simulink model "AxleSplitHEVv6_modif2019"  (R2018b)
settings: Solver=ode5  StartTime=0.0  StopTime=400  FixedStep=hev_dt  MaxStep=0.01  RelTol=1e-3  AbsTol=1e-3  EnableMultiTasking=on
PostLoadFcn:
  | load('AxelSplitHEVv4_NEDC_18_06_15.mat')
values from neighbouring files (symbols this model uses):
  cmd_equivalent_conso_coef = 0.11126984    [AxelSplitHEVv4_NEDC_18_06_15.mat]
  cmd_qmax = 42    [AxelSplitHEVv4_NEDC_18_06_15.mat]
  cmd_specific_volume_l_per_g = 0.00133333333333    [AxelSplitHEVv4_NEDC_18_06_15.mat]
  dri_cycle_speed_sp = [0 0 0 4.16666667 4.16666667 2.777777778 0 0 0 4.166666667 4.166666667 8.88888889 ... (135 elements, 135x1)]    [AxelSplitHEVv4_NEDC_18_06_15.mat]
  dri_cycle_speed_time = [0 6 11 15 23 25 28 44 49 54 56 61 ... (135 elements, 135x1)]    [AxelSplitHEVv4_NEDC_18_06_15.mat]
  dri_gbx_sp = [0 1 0 1 2 0 1 2 3 2 0 1 ... (52 elements, 52x1)]    [AxelSplitHEVv4_NEDC_18_06_15.mat]
  dri_gbx_time = [0 11 25 49 55 93 117 123 134 177 185 206 ... (52 elements, 52x1)]    [AxelSplitHEVv4_NEDC_18_06_15.mat]
  dri_ki = 24.5    [AxelSplitHEVv4_NEDC_18_06_15.mat]
  dri_kp = 609    [AxelSplitHEVv4_NEDC_18_06_15.mat]
  fa_clu_pos = [1 1 0.7 0.5 0.3 0 0]    [AxelSplitHEVv4_NEDC_18_06_15.mat]
  fa_clu_pv = [0 0.1 0.3 0.5 0.7 0.9 1]    [AxelSplitHEVv4_NEDC_18_06_15.mat]
  fa_conso_idle = 0.153611111111    [AxelSplitHEVv4_NEDC_18_06_15.mat]
  fa_conso_speed = [200 300 400 500 600 700 800 900 1000 1100 1200 1300 ... (56 elements, 1x56)]    [AxelSplitHEVv4_NEDC_18_06_15.mat]
  fa_conso_torque = [0 6.66666666667 13.3333333333 20 26.6666666667 33.3333333333 40 46.6666666667 53.3333333333 60 66.6666666667 73.3333333333 ... (43 elements, 1x43)]    [AxelSplitHEVv4_NEDC_18_06_15.mat]
  fa_delta_derating = 500    [AxelSplitHEVv4_NEDC_18_06_15.mat]
  fa_differential_ratio = FDR.fa_differential_ratio    [Algorithme_eff.m]    (also in AxelSplitHEVv4_NEDC_18_06_15.mat = 3.72; fa_differential_ratio.mat = 3.72)
  fa_fuel_consumption = [nan nan nan nan nan nan nan nan nan nan nan nan ... (2408 elements, 43x56)]    [AxelSplitHEVv4_NEDC_18_06_15.mat]    (also in Curve_fitting_conso.m = fa_fuel_consumption/max(max(fa_fuel_consumption)))
  fa_gearbox_efficiency = 0.92    [AxelSplitHEVv4_NEDC_18_06_15.mat]
  fa_gearbox_ratio = FGR.fa_gearbox_ratio    [Algorithme_eff.m]    (also in AxelSplitHEVv4_NEDC_18_06_15.mat = [0 3.98 2.21 1.47 1.1 0.89 0.75]; fa_gearbox_ratio.mat = [0 3.98 2.21 1.47 1.1 0.89 0.75])
  fa_high_derating_point = 5700    [AxelSplitHEVv4_NEDC_18_06_15.mat]
  fa_ice_inertia = 0.058    [AxelSplitHEVv4_NEDC_18_06_15.mat]
  fa_kp_idle_tr_off = 0.116198282851    [AxelSplitHEVv4_NEDC_18_06_15.mat]
  fa_kp_idle_tr_on = [1 0.8653 2.8063 6.3428 11.3274 17.3036 24.3665]    [AxelSplitHEVv4_NEDC_18_06_15.mat]
  fa_low_derating_point = 4000    [AxelSplitHEVv4_NEDC_18_06_15.mat]
  fa_max_tq_clu = 206    [AxelSplitHEVv4_NEDC_18_06_15.mat]
  fa_max_tq_ice = [0 220 233.333333333 240 246.666666667 253.333333333 253.333333333 253.333333333 260 260 266.666666667 266.666666667 ... (52 elements, 1x52)]    [AxelSplitHEVv4_NEDC_18_06_15.mat]
  fa_n_ice = [0 20 250 850 1000 1250 1500 1750 2000 2250 2500 3000 ... (18 elements, 1x18)]    [AxelSplitHEVv4_NEDC_18_06_15.mat]
  fa_starter_rpm = [0 10 20 30 40 50 60 70 80 90 100 110 ... (101 elements, 1x101)]    [AxelSplitHEVv4_NEDC_18_06_15.mat]
  fa_starter_tq = [24 24 24 24 23.3333333333 23.3333333333 23.3333333333 22.6666666667 22.6666666667 22 21.3333333333 20.6666666667 ... (101 elements, 1x101)]    [AxelSplitHEVv4_NEDC_18_06_15.mat]
  fa_tau_ice = 0.0333    [AxelSplitHEVv4_NEDC_18_06_15.mat]
  fa_taui_idle_tr_off = 0.0820482966067    [AxelSplitHEVv4_NEDC_18_06_15.mat]
  fa_taui_idle_tr_on = 0.194086623254    [AxelSplitHEVv4_NEDC_18_06_15.mat]
  fa_tq_loss = [0 -11 -10 -9 -9 -10 -11 -11 -12 -13 -14 -15 ... (18 elements, 1x18)]    [AxelSplitHEVv4_NEDC_18_06_15.mat]
  fa_tq_max_speed = [200 700 800 900 1000 1100 1200 1300 1400 1500 1600 1700 ... (52 elements, 1x52)]    [AxelSplitHEVv4_NEDC_18_06_15.mat]
  hev_dt = 0.01    [AxelSplitHEVv4_NEDC_18_06_15.mat]
  pla_csat = 1.2    [AxelSplitHEVv4_NEDC_18_06_15.mat]
  pla_equivalent_weight = 1250    [AxelSplitHEVv4_NEDC_18_06_15.mat]
  pla_f = 0.0035272    [AxelSplitHEVv4_NEDC_18_06_15.mat]
  pla_k = 0.0002318    [AxelSplitHEVv4_NEDC_18_06_15.mat]
  pla_kaero = 0.52992    [AxelSplitHEVv4_NEDC_18_06_15.mat]
  pla_max_f_brakes = 1000    [AxelSplitHEVv4_NEDC_18_06_15.mat]
  pla_wheel_radius = 0.314    [AxelSplitHEVv4_NEDC_18_06_15.mat]
  ra_electrical_machine_efficiency = [nan nan nan nan nan nan nan 91.3 91.3 91.3 91.5 91.3 ... (777 elements, 37x21)]    [AxelSplitHEVv4_NEDC_18_06_15.mat]
  ra_electrical_machine_speed = [-12000 -10800 -9600 -8400 -7200 -6000 -4800 -3600 -2400 -1200 0 1200 ... (21 elements, 1x21)]    [AxelSplitHEVv4_NEDC_18_06_15.mat]
  ra_electrical_machine_tau = 0.1    [AxelSplitHEVv4_NEDC_18_06_15.mat]
  ra_electrical_machine_torque = [-79.6460176991 -75.2212389381 -70.796460177 -66.3716814159 -61.9469026549 -57.5221238938 -53.0973451327 -48.6725663717 -44.2477876106 -39.8230088496 -35.3982300885 -30.9734513274 ... (37 elements, 1x37)]    [AxelSplitHEVv4_NEDC_18_06_15.mat]
  ra_em_max_tq = [39.8230088496 44.2477876106 53.0973451327 57.5221238938 70.796460177 79.6460176991 79.6460176991 79.6460176991 79.6460176991 79.6460176991 79.6460176991 79.6460176991 ... (21 elements, 1x21)]    [AxelSplitHEVv4_NEDC_18_06_15.mat]
  ra_em_min_tq = [-39.8230088496 -44.2477876106 -53.0973451327 -57.5221238938 -70.796460177 -79.6460176991 -79.6460176991 -79.6460176991 -79.6460176991 -79.6460176991 -79.6460176991 -79.6460176991 ... (21 elements, 1x21)]    [AxelSplitHEVv4_NEDC_18_06_15.mat]
  ra_transmission_efficiency = 0.92    [AxelSplitHEVv4_NEDC_18_06_15.mat]
  reducteur = 2    [Main_modif.m]
  syse_aux_current = 33.3    [AxelSplitHEVv4_NEDC_18_06_15.mat]
  syse_aux_voltage = 12    [AxelSplitHEVv4_NEDC_18_06_15.mat]
  syse_bat_nominal_capacity_as = 151200    [AxelSplitHEVv4_NEDC_18_06_15.mat]
  syse_cdl = 5000    [AxelSplitHEVv4_NEDC_18_06_15.mat]
  syse_dcdc_efficency = [78 89.6 92.5 95.2 95 94.6]    [AxelSplitHEVv4_NEDC_18_06_15.mat]
  syse_dcdc_in_power = [54 135 202 405 1485 2000]    [AxelSplitHEVv4_NEDC_18_06_15.mat]
  syse_electrical_machine_torque_vs_power_speed_nneg = [38.4209635438 42.3166718474 53.0973451327 53.8788373627 63.500986907 77.9700595469 78.3175021924 76.9635177026 72.2987813984 47.9837613501 38.4209635438 42.3166718474 ... (220 elements, 10x22)]    [AxelSplitHEVv4_NEDC_18_06_15.mat]
  syse_electrical_machine_torque_vs_power_speed_npos = [-72.2987813984 -76.9635177026 -78.3175021924 -77.9700595469 -63.500986907 -53.8788373627 -53.0973451327 -42.3166718474 -38.4209635438 -72.2987813984 -76.9635177026 -78.3175021924 ... (198 elements, 9x22)]    [AxelSplitHEVv4_NEDC_18_06_15.mat]
  syse_em_in_power = [-49.1089315336 -44.1089315336 -39.1089315336 -34.1089315336 -29.1089315336 -24.1089315336 -19.1089315336 -14.1089315336 -9.10893153364 -4.10893153364 0.891068466363 5.89106846636 ... (22 elements, 1x22)]    [AxelSplitHEVv4_NEDC_18_06_15.mat]
  syse_max_charge_current = [8.4 8.4 42 92.4 92.4 92.4 92.4 92.4 79.8 42 21 4.2]    [AxelSplitHEVv4_NEDC_18_06_15.mat]
  syse_max_discharge_current = [42 42 79.8 159.6 180.6 180.6 180.6 180.6 180.6 180.6 180.6 180.6]    [AxelSplitHEVv4_NEDC_18_06_15.mat]
  syse_nb_cell = 52    [AxelSplitHEVv4_NEDC_18_06_15.mat]
  syse_rdl = 0.004    [AxelSplitHEVv4_NEDC_18_06_15.mat]
  syse_rser = 0.002    [AxelSplitHEVv4_NEDC_18_06_15.mat]
  syse_soc_current_limits = [0 10 20 20.1 30 40 50 60 70 80 90 100]    [AxelSplitHEVv4_NEDC_18_06_15.mat]
  syse_soc_initial = 0.8    [AxelSplitHEVv4_NEDC_18_06_15.mat]
  syse_soc_ocv = [0 5 10 20 40 50 60 70 80 90 100]    [AxelSplitHEVv4_NEDC_18_06_15.mat]
  syse_vocv = [2.5 3.2135 3.5127 3.66 3.7771 3.8181 3.8686 3.8978 3.9429 4.0006 4.198]    [AxelSplitHEVv4_NEDC_18_06_15.mat]
undefined symbols (not defined in the file or in its folder): DiscIntNeverNeededParam
libraries: simulink x23, simulink_extras x1
(part 1 of 3)
settings Model: Creator=jboursie  LastModifiedBy=test
settings SolverCC: AutoScaleAbsTol=off  AlgebraicLoopSolver=LineSearch
settings DataIOCC: SaveFormat=Array  SignalLoggingSaveFormat=ModelDataLogs  SaveOutput=off  SignalLogging=off  DSMLogging=off  SaveTime=off
settings OptimizationCC: LifeSpan=inf
settings DebuggingCC: AlgebraicLoopMsg=error  UnderspecifiedInitializationDetection=Classic  MergeDetectMultiDrivingBlocksExec=none  SolverPrmCheckMsg=warning  MultiTaskCondExecSysMsg=none  MultiTaskRateTransMsg=warning  FcnCallInpInsideContextMsg=warning  BusObjectLabelMismatch=error  StateNameClashWarn=warning  SFUnexpectedBacktrackingDiag=warning  SFNoUnconditionalDefaultTransitionDiag=warning  SFExecutionAtInitializationDiag=none
settings HardwareCC: ProdBitPerPointer=32  ProdBitPerSizeT=32  ProdBitPerPtrDiffT=32  ProdLargestAtomicFloat=None  ProdIntDivRoundTo=Undefined  ProdEndianess=Unspecified  ProdWordSize=32  ProdHWDeviceType=32-bit Generic
settings ModelReferenceCC: PropagateSignalLabelsOutOfModel=off
settings SFSimCC: SimUseLocalCustomCode=off
settings RTWCC: RTWUseLocalCustomCode=off
settings CodeAppCC: StateflowObjectComments=on
settings GRTTargetCC: TargetLangStandard=C89/C90 (ANSI)  GeneratePreprocessorConditionals=Disable all  CombineOutputUpdateFcns=off  GRTInterface=on
settings ConfigComp: CovMetricSettings=dw  CovHtmlReporting=on  CovSaveCumulativeToWorkspaceVar=on  CovSaveSingleToWorkspaceVar=on  CovExternalEMLEnable=off

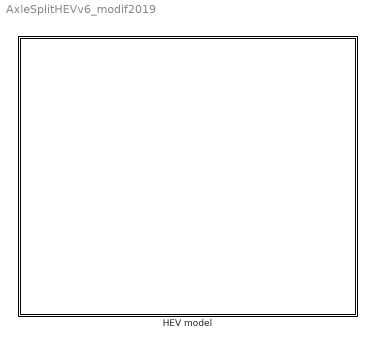
== system AxleSplitHEVv6_modif2019 ==
  HEV model : Subsystem

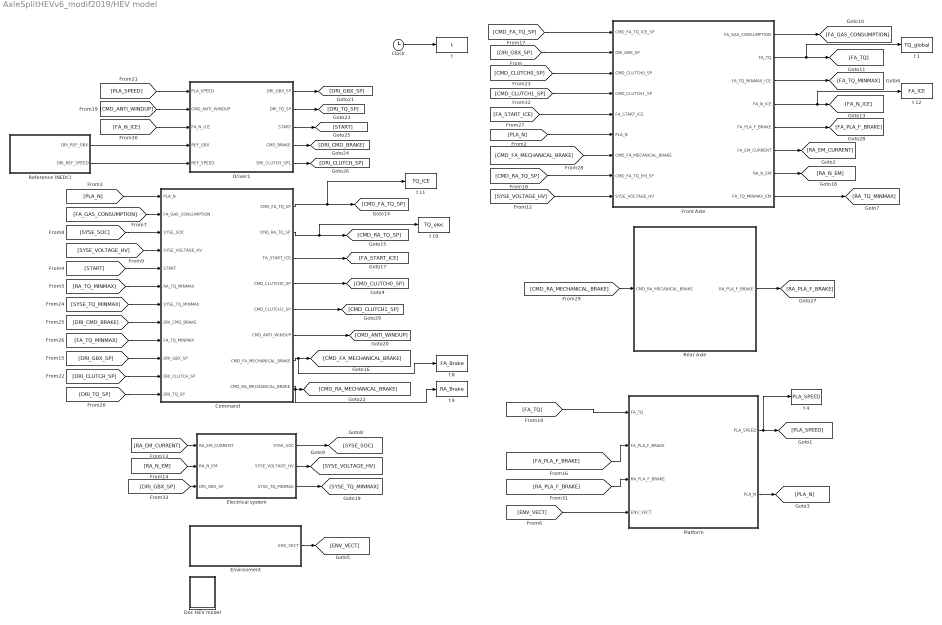
== system AxleSplitHEVv6_modif2019/HEV model ==
  Clock : Clock
  Command : Subsystem
  Doc HEV model : Subsystem
      settings: OpenFcn=open('Documents\HEVmodel.pdf')
      mask Display: fprintf('DOC')
  Driver1 : Subsystem
  Electrical system : Subsystem
  Environment : Subsystem
  Front Axle : Subsystem
  Platform : Subsystem
  Rear Axle : Subsystem
  Reference (NEDC) : Subsystem
  "t " : ToWorkspace  VariableName=t  SampleTime=hev_dt
  t 1 : ToWorkspace  VariableName=TQ_global  SampleTime=hev_dt
  t 10 : ToWorkspace  VariableName=TQ_elec  SampleTime=hev_dt
  t 11 : ToWorkspace  VariableName=TQ_ICE  SampleTime=hev_dt
  t 12 : ToWorkspace  VariableName=FA_ICE  SampleTime=hev_dt
  t 4 : ToWorkspace  VariableName=PLA_SPEED  SampleTime=hev_dt
  t 8 : ToWorkspace  VariableName=FA_Brake  SampleTime=hev_dt
  t 9 : ToWorkspace  VariableName=RA_Brake  SampleTime=hev_dt
  wires:
  Environment/1(ENV_VECT) -> [ENV_VECT]
  Electrical system/2(SYSE_VOLTAGE_HV) -> [SYSE_VOLTAGE_HV]
  Electrical system/1(SYSE_SOC) -> [SYSE_SOC]
  [RA_EM_CURRENT] -> Electrical system/1(RA_EM_CURRENT)
  [RA_N_EM] -> Electrical system/2(RA_N_EM)
  Electrical system/3(SYSE_TQ_MINMAX) -> [SYSE_TQ_MINMAX]
  Clock/1 -> "t "/1
  [CMD_ANTI_WINDUP] -> Driver1/2(CMD_ANTI_WINDUP)
  Driver1/1(DRI_GBX_SP) -> [DRI_GBX_SP]
  Driver1/2(DRI_TQ_SP) -> [DRI_TQ_SP]
  Driver1/5(DRI_CLUTCH_SP1) -> [DRI_CLUTCH_SP]
  Driver1/3(START) -> [START]
  Driver1/4(CMD_BRAKE) -> [DRI_CMD_BRAKE]
  [FA_N_ICE] -> Driver1/3(FA_N_ICE)
  Reference (NEDC)/2(DRI_REF_SPEED) -> Driver1/5(REF_SPEED)
  Reference (NEDC)/1(DRI_REF_GBX) -> Driver1/4(REF_GBX)
  [PLA_SPEED] -> Driver1/1(PLA_SPEED)
  [PLA_N] -> Command/1(PLA_N)
  [RA_TQ_MINMAX] -> Command/6(RA_TQ_MINMAX)
  [FA_GAS_CONSUMPTION] -> Command/2(FA_GAS_CONSUMPTION)
  [SYSE_SOC] -> Command/3(SYSE_SOC)
  [SYSE_VOLTAGE_HV] -> Command/4(SYSE_VOLTAGE_HV)
  Command/2(CMD_RA_TQ_SP) -> t 10/1, [CMD_RA_TQ_SP]
  Command/7(CMD_FA_MECHANICAL_BRAKE) -> t 8/1, [CMD_FA_MECHANICAL_BRAKE]
  [DRI_TQ_SP] -> Command/12(DRI_TQ_SP)
  [DRI_CLUTCH_SP] -> Command/11(DRI_CLUTCH_SP)
  [DRI_GBX_SP] -> Command/10(DRI_GBX_SP)
  [SYSE_TQ_MINMAX] -> Command/7(SYSE_TQ_MINMAX)
  [START] -> Command/5(START)
  Command/3(FA_START_ICE) -> [FA_START_ICE]
  [DRI_CMD_BRAKE] -> Command/8(DRI_CMD_BRAKE)
  [FA_TQ_MINMAX] -> Command/9(FA_TQ_MINMAX)
  Command/4("CMD_CLUTCH0_SP ") -> [CMD_CLUTCH0_SP]
  Command/6(CMD_ANTI_WINDUP) -> [CMD_ANTI_WINDUP]
  Platform/1(PLA_SPEED) -> t 4/1, [PLA_SPEED]
  Platform/2(PLA_N) -> [PLA_N]
  Front Axle/3(FA_TQ_MINMAX_ICE) -> [FA_TQ_MINMAX]
  Front Axle/8(FA_TQ_MINMAX_EM) -> [RA_TQ_MINMAX]
  [ENV_VECT] -> Platform/4(ENV_VECT)
  Front Axle/1(FA_GAS_CONSUMPTION) -> [FA_GAS_CONSUMPTION]
  Front Axle/2(FA_TQ) -> t 1/1, [FA_TQ]
  [FA_TQ] -> Platform/1(FA_TQ)
  [SYSE_VOLTAGE_HV] -> Front Axle/9(SYSE_VOLTAGE_HV)
  Front Axle/6(FA_EM_CURRENT) -> [RA_EM_CURRENT]
  [FA_PLA_F_BRAKE] -> Platform/2(FA_PLA_F_BRAKE)
  [CMD_RA_TQ_SP] -> Front Axle/8(CMD_FA_TQ_EM_SP)
  Front Axle/7(RA_N_EM) -> [RA_N_EM]
  [PLA_N] -> Front Axle/6(PLA_N)
  [FA_START_ICE] -> Front Axle/5(FA_START_ICE)
  [DRI_GBX_SP] -> Front Axle/2(DRI_GBX_SP)
  [CMD_CLUTCH0_SP] -> Front Axle/3(CMD_CLUTCH0_SP)
  Front Axle/4(FA_N_ICE) -> t 12/1, [FA_N_ICE]
  [CMD_FA_TQ_SP] -> Front Axle/1(CMD_FA_TQ_ICE_SP)
  [CMD_FA_MECHANICAL_BRAKE] -> Front Axle/7(CMD_FA_MECANICAL_BRAKE)
  [CMD_RA_MECHANICAL_BRAKE] -> Rear Axle/1(CMD_RA_MECANICAL_BRAKE)
  [RA_PLA_F_BRAKE] -> Platform/3(RA_PLA_F_BRAKE)
  Rear Axle/1(RA_PLA_F_BRAKE) -> [RA_PLA_F_BRAKE]
  Front Axle/5(FA_PLA_F_BRAKE) -> [FA_PLA_F_BRAKE]
  Command/8(CMD_RA_MECHANICAL_BRAKE) -> t 9/1, [CMD_RA_MECHANICAL_BRAKE]
  Command/1(CMD_FA_TQ_SP) -> t 11/1, [CMD_FA_TQ_SP]
  [CMD_CLUTCH1_SP] -> Front Axle/4(CMD_CLUTCH1_SP)
  Command/5("CMD_CLUTCH1_SP ") -> [CMD_CLUTCH1_SP]
  [DRI_GBX_SP] -> Electrical system/3(DRI_GBX_SP)

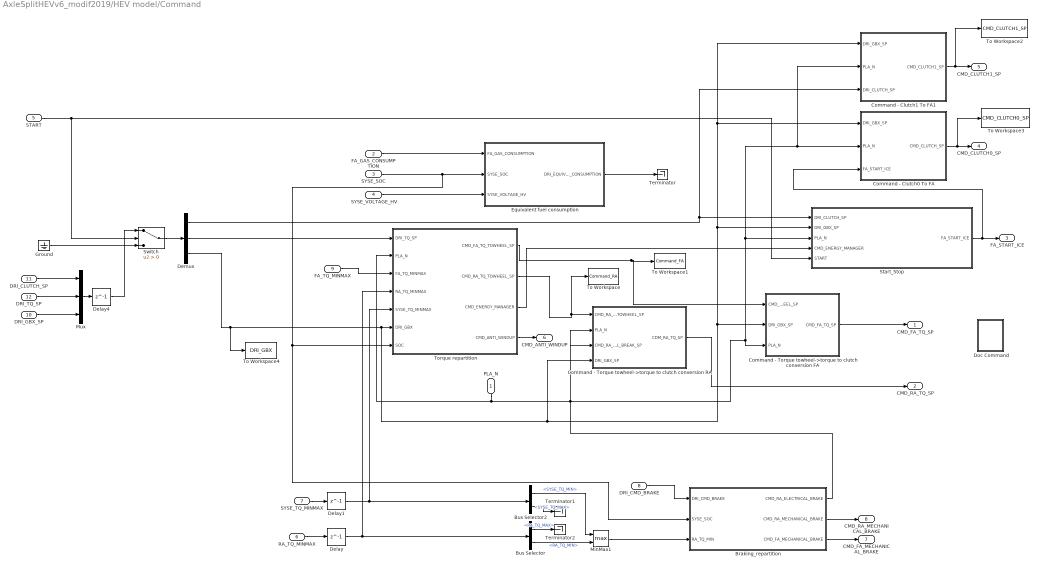
== system AxleSplitHEVv6_modif2019/HEV model/Command ==
  PLA_N : Inport
  FA_GAS_CONSUMPTION : Inport  Port=2
  SYSE_SOC : Inport  Port=3
  SYSE_VOLTAGE_HV : Inport  Port=4
  START : Inport  Port=5
  RA_TQ_MINMAX : Inport  Port=6
  SYSE_TQ_MINMAX : Inport  Port=7
  DRI_CMD_BRAKE : Inport  Port=8
  FA_TQ_MINMAX : Inport  Port=9
  DRI_GBX_SP : Inport  Port=10
  DRI_CLUTCH_SP : Inport  Port=11
  DRI_TQ_SP : Inport  Port=12
  Braking_repartition : Subsystem
  Bus Selector : BusSelector  OutputSignals=RA_TQ_MAX,RA_TQ_MIN
  Bus Selector2 : BusSelector  OutputSignals=SYSE_TQ_MIN,SYSE_TQ_MAX
  Command - Clutch0 To FA : Subsystem
  Command - Clutch1 To FA1 : Subsystem
  Command - Torque towheel->torque to clutch conversion FA : Subsystem
  Command - Torque towheel->torque to clutch conversion RA : Subsystem
  Delay : Delay  DelayLength=1
  Delay1 : Delay  DelayLength=1
  Delay4 : Delay  DelayLength=1
  Demux : Demux  Outputs=3
  Doc Command : Subsystem
      settings: OpenFcn=open('Documents\Command.pdf')
      mask Display: fprintf('DOC')
  Equivalent fuel consumption : Subsystem
  Ground : Ground
  MinMax1 : MinMax  Function=max  Inputs=2  SampleTime=hev_dt
  Mux : Mux  Inputs=3
  Start_Stop : Subsystem
  Switch : Switch  Criteria=u2 > Threshold
  Terminator : Terminator
  Terminator1 : Terminator
  Terminator2 : Terminator
  To Workspace : ToWorkspace  VariableName=Command_RA  SampleTime=-1
  To Workspace1 : ToWorkspace  VariableName=Command_FA  SampleTime=-1
  To Workspace2 : ToWorkspace  VariableName=CMD_CLUTCH1_SP  SampleTime=-1
  To Workspace3 : ToWorkspace  VariableName=CMD_CLUTCH0_SP  SampleTime=-1
  To Workspace4 : ToWorkspace  VariableName=DRI_GBX  SampleTime=-1
  Torque repartition : Subsystem
  CMD_FA_TQ_SP : Outport
  CMD_RA_TQ_SP : Outport  Port=2
  FA_START_ICE : Outport  Port=3
  "CMD_CLUTCH0_SP " : Outport  Port=4
  "CMD_CLUTCH1_SP " : Outport  Port=5
  CMD_ANTI_WINDUP : Outport  Port=6
  CMD_FA_MECHANICAL_BRAKE : Outport  Port=7
  CMD_RA_MECHANICAL_BRAKE : Outport  Port=8
  wires:
  FA_GAS_CONSUMPTION/1 -> Equivalent fuel consumption/1(FA_GAS_CONSUMPTION)
  SYSE_SOC/1 -> Equivalent fuel consumption/2(SYSE_SOC), Braking_repartition/2(SYSE_SOC), Torque repartition/7(SOC)
  SYSE_VOLTAGE_HV/1 -> Equivalent fuel consumption/3(SYSE_VOLTAGE_HV)
  Torque repartition/1(CMD_FA_TQ_TOWHEEL_SP) -> To Workspace1/1, Command - Torque towheel->torque to clutch conversion FA/1(CMD_FA_TQ_TOWHEEL_SP)
  Equivalent fuel consumption/1(DRI_EQUIV_GAZ_CONSUMPTION) -> Terminator/1
  Command - Torque towheel->torque to clutch conversion FA/1(CMD_FA_TQ_SP) -> CMD_FA_TQ_SP/1
  RA_TQ_MINMAX/1 -> Delay/1
  SYSE_TQ_MINMAX/1 -> Delay1/1
  Bus Selector2/1 -> MinMax1/1  "<SYSE_TQ_MIN>"
  Bus Selector/2 -> MinMax1/2  "<RA_TQ_MIN>"
  Bus Selector/1 -> Terminator2/1  "<RA_TQ_MAX>"
  Bus Selector2/2 -> Terminator1/1  "<SYSE_TQ_MAX>"
  Command - Torque towheel->torque to clutch conversion RA/1(CDM_RA_TQ_SP) -> CMD_RA_TQ_SP/1
  Torque repartition/2(CMD_RA_TQ_TOWHEEL_SP) -> Command - Torque towheel->torque to clutch conversion RA/1(CMD_RA_TQ_TOWHEEL_SP), To Workspace/1
  START/1 -> Start_Stop/5(START), Switch/2
  Start_Stop/1(FA_START_ICE) -> Command - Clutch0 To FA/3(FA_START_ICE), FA_START_ICE/1
  DRI_CMD_BRAKE/1 -> Braking_repartition/1(DRI_CMD_BRAKE)
  MinMax1/1 -> Braking_repartition/3(RA_TQ_MIN)
  FA_TQ_MINMAX/1 -> Torque repartition/3(FA_TQ_MINMAX)
  Delay/1 -> Bus Selector/1, Torque repartition/4(RA_TQ_MINMAX)
  Delay1/1 -> Bus Selector2/1, Torque repartition/5(SYSE_TQ_MINMAX)
  PLA_N/1 -> Command - Torque towheel->torque to clutch conversion RA/2(PLA_N), Start_Stop/3(PLA_N), Command - Clutch1 To FA1/2(PLA_N), Command - Clutch0 To FA/2(PLA_N), Command - Torque towheel->torque to clutch conversion FA/3(PLA_N), Torque repartition/2(PLA_N)
  Command - Clutch0 To FA/1("CMD_CLUTCH_SP ") -> To Workspace3/1, "CMD_CLUTCH0_SP "/1
  Torque repartition/3(CMD_ENERGY_MANAGER) -> Start_Stop/4(CMD_ENERGY_MANAGER)
  Torque repartition/4(CMD_ANTI_WINDUP) -> CMD_ANTI_WINDUP/1
  Switch/1 -> Demux/1
  DRI_GBX_SP/1 -> Mux/3
  Mux/1 -> Delay4/1
  Demux/3 -> To Workspace4/1, Command - Torque towheel->torque to clutch conversion RA/4(DRI_GBX_SP), Start_Stop/2(DRI_GBX_SP), Command - Clutch0 To FA/1(DRI_GBX_SP), Command - Clutch1 To FA1/1(DRI_GBX_SP), Command - Torque towheel->torque to clutch conversion FA/2(DRI_GBX_SP), Torque repartition/6(DRI_GBX)
  Delay4/1 -> Switch/1
  Ground/1 -> Switch/3
  DRI_CLUTCH_SP/1 -> Mux/1
  DRI_TQ_SP/1 -> Mux/2
  Demux/2 -> Torque repartition/1(DRI_TQ_SP)
  Braking_repartition/1(CMD_RA_ELECTRICAL_BRAKE) -> Command - Torque towheel->torque to clutch conversion RA/3(CMD_RA_TQ_TOWHEEL_BREAK_SP)
  Braking_repartition/3(CMD_FA_MECHANICAL_BRAKE) -> CMD_FA_MECHANICAL_BRAKE/1
  Braking_repartition/2(CMD_RA_MECHANICAL_BRAKE) -> CMD_RA_MECHANICAL_BRAKE/1
  Command - Clutch1 To FA1/1("CMD_CLUTCH1_SP ") -> To Workspace2/1, "CMD_CLUTCH1_SP "/1
  Demux/1 -> Start_Stop/1(DRI_CLUTCH_SP), Command - Clutch1 To FA1/3(DRI_CLUTCH_SP)

== system AxleSplitHEVv6_modif2019/HEV model/Doc HEV model ==

== system AxleSplitHEVv6_modif2019/HEV model/Driver1 ==
  note: Nouvelle commande START pour éveiller le système : Le conducteur ne peut démarrer le véhicule que si START est à 1
  PLA_SPEED : Inport
  CMD_ANTI_WINDUP : Inport  Port=2
  FA_N_ICE : Inport  Port=3
  REF_GBX : Inport  Port=4
  REF_SPEED : Inport  Port=5
  Clutch command : Subsystem
  Delay : Delay  DelayLength=1
  Doc Driver : Subsystem
      settings: OpenFcn=open('Documents\Driver.pdf')
      mask Display: fprintf('DOC')
  Driver : Subsystem
  Product : Product
  Step1 : Step  Time=0  SampleTime=0
  Sum2 : Sum  Inputs=-|+  SampleTime=hev_dt
  To Workspace : ToWorkspace  VariableName=DRI_TQ  SaveFormat=Timeseries  SampleTime=-1
  DRI_GBX_SP : Outport
  DRI_TQ_SP : Outport  Port=2
  START : Outport  Port=3
  CMD_BRAKE : Outport  Port=4
  DRI_CLUTCH_SP1 : Outport  Port=5
  wires:
  CMD_ANTI_WINDUP/1 -> Driver/1(CMD_ANTI_WINDUP)
  REF_GBX/1 -> Clutch command/1(DRI_REF_GBX)
  REF_SPEED/1 -> Sum2/2  "Speed_reference_km/h"
  Driver/1(DRI_TQ_SP) -> To Workspace/1, DRI_TQ_SP/1
  Driver/2(CMD_BRAKE) -> CMD_BRAKE/1
  Sum2/1 -> Driver/2(DRI_DELTA_SPEED)
  PLA_SPEED/1 -> Sum2/1
  Step1/1 -> START/1
  FA_N_ICE/1 -> Delay/1
  Clutch command/1(DRI_GBX_SP) -> DRI_GBX_SP/1
  Clutch command/2(DRI_CLUTCH_SP) -> Product/2
  Delay/1 -> Clutch command/2(FA_N_ICE)
  Driver/3(DRI_CLUTCH) -> Product/1
  Product/1 -> DRI_CLUTCH_SP1/1

== system AxleSplitHEVv6_modif2019/HEV model/Electrical system ==
  RA_EM_CURRENT : Inport
  RA_N_EM : Inport  Port=2
  DRI_GBX_SP : Inport  Port=3
  Add : Sum  SampleTime=hev_dt
  Auxiliary network 12V : Subsystem
  Bus Creator : BusCreator  Inputs=2
  Delay : Delay  DelayLength=1  SampleTime=hev_dt
  Doc Electrical system : Subsystem
      settings: OpenFcn=open('Documents\ElectricalSystem.pdf')
      mask Display: fprintf('DOC')
  Electrical System supervision : Subsystem
  Lithium-Ion Battery Management System : Subsystem
  SYSE_SOC : Outport
  SYSE_VOLTAGE_HV : Outport  Port=2
  SYSE_TQ_MINMAX : Outport  Port=3
  wires:
  Add/1 -> Delay/1  "A"
  Lithium-Ion Battery Management System/2(SYSE_VOLTAGE_HV) -> Electrical System supervision/4(SYSE_VOLTAGE_HV), SYSE_VOLTAGE_HV/1, Auxiliary network 12V/1(SYSE_VOLTAGE_HV)  "V"
  Lithium-Ion Battery Management System/1(SYSE_SOC) -> SYSE_SOC/1, Electrical System supervision/2(SYSE_SOC)
  Electrical System supervision/2(SYSE_TQ_MIN) -> Bus Creator/2  "SYSE_TQ_MIN"
  Electrical System supervision/1(SYSE_TQ_MAX) -> Bus Creator/1  "SYSE_TQ_MAX"
  RA_EM_CURRENT/1 -> Add/1
  RA_N_EM/1 -> Electrical System supervision/1(RA_N_EM)
  Auxiliary network 12V/1(SYSE_AUX_CURRENT) -> Electrical System supervision/3(SYSE_AUX_CURRENT), Add/2  "A"
  Delay/1 -> Lithium-Ion Battery Management System/1(SYSE_LIION_CURRENT)
  Bus Creator/1 -> SYSE_TQ_MINMAX/1
  DRI_GBX_SP/1 -> Electrical System supervision/5(DRI_GBX_SP)

== system AxleSplitHEVv6_modif2019/HEV model/Environment ==
  Bus Creator : BusCreator  Inputs=3
  Constant : Constant  Value=0
  Constant1 : Constant  Value=0
  Constant2 : Constant  Value=0
  ENV_VECT : Outport
  wires:
  Constant2/1 -> Bus Creator/1  "Slope[%]"
  Constant/1 -> Bus Creator/2  "F_ext"
  Constant1/1 -> Bus Creator/3  "Wind"
  Bus Creator/1 -> ENV_VECT/1  "Environment"

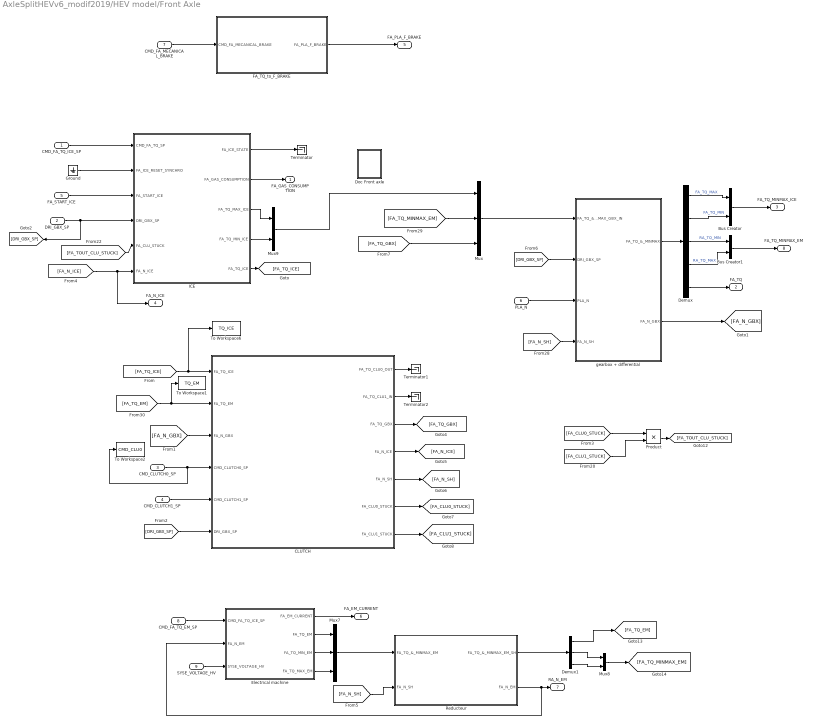
== system AxleSplitHEVv6_modif2019/HEV model/Front Axle ==
  CMD_FA_TQ_ICE_SP : Inport
  DRI_GBX_SP : Inport  Port=2
  CMD_CLUTCH0_SP : Inport  Port=3
  CMD_CLUTCH1_SP : Inport  Port=4
  FA_START_ICE : Inport  Port=5
  PLA_N : Inport  Port=6
  CMD_FA_MECANICAL_BRAKE : Inport  Port=7
  CMD_FA_TQ_EM_SP : Inport  Port=8
  SYSE_VOLTAGE_HV : Inport  Port=9
  Bus Creator : BusCreator  Inputs=2
  Bus Creator1 : BusCreator  Inputs=2
  CLUTCH : Subsystem
  Demux : Demux  Outputs=5
  Demux1 : Demux  Outputs=3
  Doc Front axle : Subsystem
      settings: OpenFcn=open('Documents\FrontAxle.pdf')
      mask Display: fprintf('DOC')
  Electrical machine : Subsystem
  FA_TQ_to_F_BRAKE : Subsystem
  Ground : Ground
  ICE : Subsystem
  Mux : Mux  Inputs=3
  Mux7 : Mux  Inputs=3
  Mux8 : Mux  Inputs=2
  Mux9 : Mux  Inputs=2
  Product : Product
  Reducteur : Subsystem
  Terminator : Terminator
  Terminator1 : Terminator
  Terminator2 : Terminator
  To Workspace1 : ToWorkspace  VariableName=TQ_EM  SampleTime=-1
  To Workspace2 : ToWorkspace  VariableName=CMD_CLU0  SampleTime=-1
  To Workspace6 : ToWorkspace  VariableName=TQ_ICE  SampleTime=-1
  gearbox + differential : Subsystem
  FA_GAS_CONSUMPTION : Outport
  FA_TQ : Outport  Port=2
  FA_TQ_MINMAX_ICE : Outport  Port=3
  FA_N_ICE : Outport  Port=4
  FA_PLA_F_BRAKE : Outport  Port=5
  FA_EM_CURRENT : Outport  Port=6
  RA_N_EM : Outport  Port=7
  FA_TQ_MINMAX_EM : Outport  Port=8
  wires:
  Bus Creator/1 -> FA_TQ_MINMAX_ICE/1
  Mux/1 -> gearbox + differential/1(FA_TQ_&_MINMAX_GBX_IN)
  ICE/2(FA_GAS_CONSUMPTION) -> FA_GAS_CONSUMPTION/1
  ICE/1(FA_ICE_STATE) -> Terminator/1
  Demux/1 -> Bus Creator/1  "FA_TQ_MAX"
  Demux/2 -> Bus Creator/2  "FA_TQ_MIN"
  DRI_GBX_SP/1 -> ICE/4(DRI_GBX_SP), [DRI_GBX_SP]
  Ground/1 -> ICE/2(FA_ICE_RESET_SYNCHRO)
  PLA_N/1 -> gearbox + differential/3(PLA_N)
  CMD_FA_TQ_ICE_SP/1 -> ICE/1(CMD_FA_TQ_SP)
  CMD_FA_MECANICAL_BRAKE/1 -> FA_TQ_to_F_BRAKE/1(CMD_FA_MECANICAL_BRAKE)
  FA_TQ_to_F_BRAKE/1(FA_PLA_F_BRAKE) -> FA_PLA_F_BRAKE/1
  ICE/5(FA_TQ_ICE) -> [FA_TQ_ICE]
  [FA_TQ_ICE] -> To Workspace6/1, CLUTCH/1(FA_TQ_ICE)
  gearbox + differential/2(FA_N_GBX) -> [FA_N_GBX]
  [FA_N_GBX] -> CLUTCH/3(FA_N_GBX)
  [FA_TQ_EM] -> To Workspace1/1, CLUTCH/2(FA_TQ_EM)
  CMD_CLUTCH1_SP/1 -> CLUTCH/5(CMD_CLUTCH1_SP)
  CMD_CLUTCH0_SP/1 -> To Workspace2/1, CLUTCH/4(CMD_CLUTCH0_SP)
  [DRI_GBX_SP] -> CLUTCH/6(DRI_GBX_SP)
  CLUTCH/7(FA_CLU1_STUCK) -> [FA_CLU1_STUCK]
  CLUTCH/3(FA_TQ_GBX) -> [FA_TQ_GBX]
  CLUTCH/6(FA_CLU0_STUCK) -> [FA_CLU0_STUCK]
  CLUTCH/4(FA_N_ICE) -> [FA_N_ICE]
  CLUTCH/5(FA_N_SH) -> [FA_N_SH]
  [FA_N_ICE] -> FA_N_ICE/1, ICE/6(FA_N_ICE)
  [DRI_GBX_SP] -> gearbox + differential/2(DRI_GBX_SP)
  [FA_CLU0_STUCK] -> Product/1
  [FA_CLU1_STUCK] -> Product/2
  Product/1 -> [FA_TOUT_CLU_STUCK]
  [FA_TOUT_CLU_STUCK] -> ICE/5(FA_CLU_STUCK)
  Electrical machine/1(FA_EM_CURRENT) -> FA_EM_CURRENT/1
  Electrical machine/3(FA_TQ_MIN_EM) -> Mux7/2
  [FA_N_SH] -> Reducteur/2(FA_N_SH)
  Reducteur/1(FA_TQ_&_MINMAX_EM_SH) -> Demux1/1
  Reducteur/2(FA_N_EM) -> Electrical machine/2(FA_N_EM), RA_N_EM/1
  Demux1/1 -> [FA_TQ_EM]
  Electrical machine/2(FA_TQ_EM) -> Mux7/1
  Electrical machine/4(FA_TQ_MAX_EM) -> Mux7/3
  SYSE_VOLTAGE_HV/1 -> Electrical machine/3(SYSE_VOLTAGE_HV)
  Mux7/1 -> Reducteur/1(FA_TQ_&_MINMAX_EM)
  CMD_FA_TQ_EM_SP/1 -> Electrical machine/1(CMD_FA_TQ_ICE_SP)
  Demux/3 -> Bus Creator1/1  "RA_TQ_MIN"
  Demux/4 -> Bus Creator1/2  "RA_TQ_MAX"
  Bus Creator1/1 -> FA_TQ_MINMAX_EM/1
  Demux1/3 -> Mux8/2
  Demux1/2 -> Mux8/1
  Mux8/1 -> [FA_TQ_MINMAX_EM]
  [FA_TQ_MINMAX_EM] -> Mux/2
  ICE/3(FA_TQ_MAX_ICE) -> Mux9/1
  ICE/4(FA_TQ_MIN_ICE) -> Mux9/2
  Mux9/1 -> Mux/1
  gearbox + differential/1(FA_TQ_&_MINMAX) -> Demux/1
  Demux/5 -> FA_TQ/1
  FA_START_ICE/1 -> ICE/3(FA_START_ICE)
  [FA_TQ_GBX] -> Mux/3
  [FA_N_SH] -> gearbox + differential/4(FA_N_SH)
  CLUTCH/2(FA_TQ_CLU1_IN) -> Terminator2/1
  CLUTCH/1(FA_TQ_CLU0_OUT) -> Terminator1/1

== system AxleSplitHEVv6_modif2019/HEV model/Platform ==
  FA_TQ : Inport
  FA_PLA_F_BRAKE : Inport  Port=2
  RA_PLA_F_BRAKE : Inport  Port=3
  ENV_VECT : Inport  Port=4
  Bus Selector : BusSelector  OutputSignals=Slope[%],F_ext,Wind
  Doc Platform : Subsystem
      settings: OpenFcn=open('Documents\Platform.pdf')
      mask Display: fprintf('DOC')
  Gain : Gain  Gain=3.6  SampleTime=hev_dt
  Mechanical behavior : Subsystem
  Sum1 : Sum  Inputs=+|+  SampleTime=hev_dt
  "m/s -> tr/min" : Gain  Gain=60/(2*pi*pla_wheel_radius)  SampleTime=hev_dt
  PLA_SPEED : Outport
  PLA_N : Outport  Port=2
  wires:
  Mechanical behavior/1(PLA_SPEED_MS) -> Gain/1, "m/s -> tr/min"/1
  ENV_VECT/1 -> Bus Selector/1
  Bus Selector/1 -> Mechanical behavior/3(ENV_SLOPE_PERCENT)  "<Slope[%]>"
  Bus Selector/2 -> Mechanical behavior/4(ENV_EXTERNAL_FORCES)  "<F_ext>"
  Bus Selector/3 -> Mechanical behavior/5(ENV_WIND_SPEED)  "<Wind>"
  Gain/1 -> PLA_SPEED/1
  "m/s -> tr/min"/1 -> PLA_N/1
  FA_TQ/1 -> Mechanical behavior/1(PLA_TQ_SUM)
  Sum1/1 -> Mechanical behavior/2(CMD_BRAKE_SP)
  RA_PLA_F_BRAKE/1 -> Sum1/2
  FA_PLA_F_BRAKE/1 -> Sum1/1

== system AxleSplitHEVv6_modif2019/HEV model/Rear Axle ==
  CMD_RA_MECANICAL_BRAKE : Inport
  Doc Rear axle : Subsystem
      settings: OpenFcn=open('Documents\RearAxle.pdf')
      mask Display: fprintf('DOC')
  RA_TQ_to_F_BRAKE : Subsystem
  RA_PLA_F_BRAKE : Outport
  wires:
  CMD_RA_MECANICAL_BRAKE/1 -> RA_TQ_to_F_BRAKE/1(CMD_RA_MECANICAL_BRAKE)
  RA_TQ_to_F_BRAKE/1(RA_PLA_F_BRAKE) -> RA_PLA_F_BRAKE/1

== system AxleSplitHEVv6_modif2019/HEV model/Reference (NEDC) ==
  Clock : Clock
  NEDC gear : Lookup_n-D  NumberOfTableDimensions=1  BreakpointsForDimension1=dri_gbx_time  Table=dri_gbx_sp  InterpMethod=Flat  SampleTime=hev_dt  RndMeth=Simplest  InputSameDT=on
  NEDC speed : Lookup_n-D  NumberOfTableDimensions=1  BreakpointsForDimension1=dri_cycle_speed_time  Table=dri_cycle_speed_sp  SampleTime=hev_dt  RndMeth=Simplest  InputSameDT=on
  Quantizer : Quantizer  QuantizationInterval=1  SampleTime=hev_dt
  To Workspace : ToWorkspace  VariableName=Boite_ref  SampleTime=-1
  To Workspace1 : ToWorkspace  VariableName=V_ref  SampleTime=-1
  "m/s -> km/h" : Gain  Gain=3.6  SampleTime=hev_dt
  DRI_REF_GBX : Outport
  DRI_REF_SPEED : Outport  Port=2
  wires:
  NEDC gear/1 -> Quantizer/1
  Quantizer/1 -> To Workspace/1, DRI_REF_GBX/1
  Clock/1 -> NEDC speed/1, NEDC gear/1
  NEDC speed/1 -> "m/s -> km/h"/1
  "m/s -> km/h"/1 -> To Workspace1/1, DRI_REF_SPEED/1

== system AxleSplitHEVv6_modif2019/HEV model/Command/Braking_repartition ==
  DRI_CMD_BRAKE : Inport
  SYSE_SOC : Inport  Port=2
  RA_TQ_MIN : Inport  Port=3
  BREAK REPARTITION FRONT/REAR : Subsystem
  BREAKE REPARTITION RA : Subsystem
  CMD_RA_ELECTRICAL_BRAKE : Outport
  CMD_RA_MECHANICAL_BRAKE : Outport  Port=2
  CMD_FA_MECHANICAL_BRAKE : Outport  Port=3
  wires:
  DRI_CMD_BRAKE/1 -> BREAK REPARTITION FRONT/REAR/1(DRI_CMD_BRAKE)
  BREAK REPARTITION FRONT/REAR/1(CMD_FA_BRAKE) -> CMD_FA_MECHANICAL_BRAKE/1
  BREAK REPARTITION FRONT/REAR/2(CMD_RA_BRAKE) -> BREAKE REPARTITION RA/1(CMD_RA_BREAK)
  SYSE_SOC/1 -> BREAKE REPARTITION RA/2(SYSE_SOC)
  RA_TQ_MIN/1 -> BREAKE REPARTITION RA/3(RA_TQ_MIN)
  BREAKE REPARTITION RA/1(CMD_RA_MECHANICAL_BRAKE) -> CMD_RA_MECHANICAL_BRAKE/1
  BREAKE REPARTITION RA/2(CMD_RA_ELECTRICAL_BRAKE) -> CMD_RA_ELECTRICAL_BRAKE/1

== system AxleSplitHEVv6_modif2019/HEV model/Command/Command - Clutch0 To FA ==
  DRI_GBX_SP : Inport
  PLA_N : Inport  Port=2
  FA_START_ICE : Inport  Port=3
  Compare To Constant : simulink/Logic and Bit Operations/Compare To Constant  relop===  const=0  OutDataTypeStr=uint8
  Compare To Constant1 : simulink/Logic and Bit Operations/Compare To Constant  relop=<=  const=0.01  OutDataTypeStr=uint8
  Constant : Constant
  Constant1 : Constant  Value=0
  Data Type Conversion : DataTypeConversion
  Ground1 : Ground
  Ground2 : Ground
  Switch2 : Switch  Criteria=u2 ~= 0  Threshold=1
  Terminator1 : Terminator
  Terminator2 : Terminator
  car stopped or open clutch : Logic  Operator=OR  Inputs=3  AllPortsSameDT=off  OutDataTypeStr=boolean
  car stopped or open clutch1 : Logic  Operator=NOT  Inputs=3  AllPortsSameDT=off  OutDataTypeStr=boolean
  "CMD_CLUTCH_SP " : Outport
  wires:
  Switch2/1 -> "CMD_CLUTCH_SP "/1
  DRI_GBX_SP/1 -> Compare To Constant/1
  Compare To Constant/1 -> Terminator1/1
  car stopped or open clutch/1 -> Switch2/2
  PLA_N/1 -> Compare To Constant1/1
  Constant/1 -> Switch2/1
  FA_START_ICE/1 -> Data Type Conversion/1
  Data Type Conversion/1 -> car stopped or open clutch1/1
  Compare To Constant1/1 -> car stopped or open clutch/1
  Ground1/1 -> car stopped or open clutch/2
  car stopped or open clutch1/1 -> car stopped or open clutch/3
  Ground2/1 -> Terminator2/1
  Constant1/1 -> Switch2/3

== system AxleSplitHEVv6_modif2019/HEV model/Command/Command - Clutch1 To FA1 ==
  DRI_GBX_SP : Inport
  PLA_N : Inport  Port=2
  DRI_CLUTCH_SP : Inport  Port=3
  Compare To Constant : simulink/Logic and Bit Operations/Compare To Constant  relop===  const=0  OutDataTypeStr=uint8
  Compare To Constant1 : simulink/Logic and Bit Operations/Compare To Constant  relop=<=  const=0.01  OutDataTypeStr=uint8
  Constant : Constant
  Ground2 : Ground
  Switch2 : Switch  Criteria=u2 ~= 0  Threshold=1
  Terminator : Terminator
  Terminator2 : Terminator
  car stopped or open clutch : Logic  Operator=OR  AllPortsSameDT=off  OutDataTypeStr=boolean
  "CMD_CLUTCH1_SP " : Outport
  wires:
  Switch2/1 -> Terminator/1
  DRI_GBX_SP/1 -> Compare To Constant/1
  car stopped or open clutch/1 -> Switch2/2
  PLA_N/1 -> Compare To Constant1/1
  Constant/1 -> Switch2/1
  Compare To Constant1/1 -> car stopped or open clutch/1
  Compare To Constant/1 -> car stopped or open clutch/2
  Ground2/1 -> Terminator2/1
  DRI_CLUTCH_SP/1 -> "CMD_CLUTCH1_SP "/1, Switch2/3

== system AxleSplitHEVv6_modif2019/HEV model/Command/Command - Torque towheel->torque to clutch conversion FA ==
  CMD_FA_TQ_TOWHEEL_SP : Inport
  DRI_GBX_SP : Inport  Port=2
  PLA_N : Inport  Port=3
  Differential ratio : Gain  Gain=fa_differential_ratio  SampleTime=hev_dt
  Divide2 : Product  Inputs=*/  SampleTime=hev_dt
  Efficiency P neg : Gain  Gain=2-fa_gearbox_efficiency  SampleTime=hev_dt
  Ground1 : Ground
  Product : Product  SampleTime=hev_dt
  Switch : Switch  SampleTime=hev_dt
  Switch1 : Switch  Criteria=u2 ~= 0  SampleTime=hev_dt
  efficiency P pos : Gain  Gain=fa_gearbox_efficiency  SampleTime=hev_dt
  gear ratio : LookupNDDirect  NumberOfTableDimensions=1  Table=fa_gearbox_ratio  SampleTime=hev_dt
  CMD_FA_TQ_SP : Outport
  wires:
  DRI_GBX_SP/1 -> gear ratio/1
  gear ratio/1 -> Differential ratio/1, Switch1/2
  Differential ratio/1 -> Divide2/2
  CMD_FA_TQ_TOWHEEL_SP/1 -> Product/2, Efficiency P neg/1, efficiency P pos/1
  efficiency P pos/1 -> Switch/1
  Efficiency P neg/1 -> Switch/3
  Product/1 -> Switch/2
  Switch/1 -> Divide2/1
  PLA_N/1 -> Product/1
  Ground1/1 -> Switch1/3
  Switch1/1 -> CMD_FA_TQ_SP/1
  Divide2/1 -> Switch1/1

== system AxleSplitHEVv6_modif2019/HEV model/Command/Command - Torque towheel->torque to clutch conversion RA ==
  CMD_RA_TQ_TOWHEEL_SP : Inport
  PLA_N : Inport  Port=2
  CMD_RA_TQ_TOWHEEL_BREAK_SP : Inport  Port=3
  DRI_GBX_SP : Inport  Port=4
  Differential ratio : Gain  Gain=1/reducteur  SampleTime=hev_dt
  Differential ratio1 : Gain  Gain=fa_differential_ratio  SampleTime=hev_dt
  Divide2 : Product  Inputs=*/  SampleTime=hev_dt
  Efficiency P neg : Gain  Gain=2-ra_transmission_efficiency  SampleTime=hev_dt
  Efficiency P neg1 : Gain  Gain=2-fa_gearbox_efficiency  SampleTime=hev_dt
  Efficiency P pos : Gain  Gain=ra_transmission_efficiency  SampleTime=hev_dt
  Ground1 : Ground
  Product : Product  SampleTime=hev_dt
  Product1 : Product  SampleTime=hev_dt
  Sum : Sum  Inputs=|+-
  Switch : Switch  SampleTime=hev_dt
  Switch1 : Switch  SampleTime=hev_dt
  Switch2 : Switch  Criteria=u2 ~= 0  SampleTime=hev_dt
  efficiency P pos : Gain  Gain=fa_gearbox_efficiency  SampleTime=hev_dt
  gear ratio : LookupNDDirect  NumberOfTableDimensions=1  Table=fa_gearbox_ratio  SampleTime=hev_dt
  CDM_RA_TQ_SP : Outport
  wires:
  CMD_RA_TQ_TOWHEEL_BREAK_SP/1 -> Sum/2
  Differential ratio/1 -> CDM_RA_TQ_SP/1
  efficiency P pos/1 -> Switch1/1
  Switch2/1 -> Product/2, Efficiency P pos/1, Efficiency P neg/1
  PLA_N/1 -> Product/1, Product1/1
  Divide2/1 -> Switch2/1
  Efficiency P neg1/1 -> Switch1/3
  CMD_RA_TQ_TOWHEEL_SP/1 -> Sum/1
  Product1/1 -> Switch1/2
  Switch1/1 -> Divide2/1
  gear ratio/1 -> Differential ratio1/1, Switch2/2
  Efficiency P neg/1 -> Switch/3
  Efficiency P pos/1 -> Switch/1
  Product/1 -> Switch/2
  Sum/1 -> Product1/2, Efficiency P neg1/1, efficiency P pos/1
  Differential ratio1/1 -> Divide2/2
  DRI_GBX_SP/1 -> gear ratio/1
  Switch/1 -> Differential ratio/1
  Ground1/1 -> Switch2/3

== system AxleSplitHEVv6_modif2019/HEV model/Command/Doc Command ==

== system AxleSplitHEVv6_modif2019/HEV model/Command/Equivalent fuel consumption ==
  FA_GAS_CONSUMPTION : Inport
  SYSE_SOC : Inport  Port=2
  SYSE_VOLTAGE_HV : Inport  Port=3
  Constant : Constant  Value=0
  Delay : Delay  DelayLength=1  SampleTime=hev_dt
  Discrete Zero-Pole : DiscreteZeroPole  Zeros=[-1]  Poles=[1]  Gain=1  SampleTime=hev_dt
  Discrete Zero-Pole1 : DiscreteZeroPole  Zeros=[-1]  Poles=[1]  Gain=1  SampleTime=hev_dt
  Gain1 : Gain  Gain=cmd_qmax  SampleTime=hev_dt
  Gain2 : Gain  Gain=0.0036  SampleTime=hev_dt
  Gain3 : Gain  Gain=0.2777777778  SampleTime=hev_dt
  Gain4 : Gain  Gain=cmd_equivalent_conso_coef  SampleTime=hev_dt
  Gain5 : Gain  Gain=cmd_specific_volume_l_per_g  SampleTime=hev_dt
  Gain6 : Gain  Gain=hev_dt/2  SampleTime=hev_dt
  Gain7 : Gain  Gain=hev_dt/2  SampleTime=hev_dt
  Product : Product  SampleTime=hev_dt
  Relational Operator : RelationalOperator  Operator=isNaN  OutDataTypeStr=boolean  SampleTime=hev_dt  RndMeth=Nearest
  Sum : Sum  Inputs=+-|  SampleTime=hev_dt
  Sum1 : Sum  Inputs=|++  SampleTime=hev_dt
  Switch : Switch  Criteria=u2 ~= 0  SampleTime=hev_dt
  DRI_EQUIV_GAZ_CONSUMPTION : Outport
  wires:
  Gain2/1 -> Gain3/1
  Product/1 -> Gain2/1
  SYSE_SOC/1 -> Delay/1, Sum/2
  Delay/1 -> Sum/1
  Sum/1 -> Gain1/1
  SYSE_VOLTAGE_HV/1 -> Product/2
  Gain3/1 -> Gain4/1
  Sum1/1 -> DRI_EQUIV_GAZ_CONSUMPTION/1
  Gain5/1 -> Sum1/1
  Discrete Zero-Pole/1 -> Sum1/2
  Gain1/1 -> Product/1
  FA_GAS_CONSUMPTION/1 -> Relational Operator/1, Switch/3
  Relational Operator/1 -> Switch/2
  Constant/1 -> Switch/1
  Gain4/1 -> Gain7/1
  Gain7/1 -> Discrete Zero-Pole/1
  Switch/1 -> Gain6/1
  Discrete Zero-Pole1/1 -> Gain5/1
  Gain6/1 -> Discrete Zero-Pole1/1

== system AxleSplitHEVv6_modif2019/HEV model/Command/Start_Stop ==
  DRI_CLUTCH_SP : Inport
  DRI_GBX_SP : Inport  Port=2
  PLA_N : Inport  Port=3
  CMD_ENERGY_MANAGER : Inport  Port=4
  START : Inport  Port=5
  Data Type Conversion : DataTypeConversion
  Delay3 : Delay  DelayLength=1
  Logical Operator : Logic  Operator=OR  AllPortsSameDT=off  OutDataTypeStr=boolean
  START/STOP 1 : Stateflow chart  TreatAsAtomicUnit=on
  startstop prototype : Subsystem
  FA_START_ICE : Outport
  wires:
  DRI_CLUTCH_SP/1 -> startstop prototype/4(DRI_CLUTCH_SP)
  PLA_N/1 -> startstop prototype/1(PLA_N)
  DRI_GBX_SP/1 -> startstop prototype/2(DRI_GBX_SP)
  START/STOP 1/2(ENERGY_MANAGEMENT_ON_OFF) -> Delay3/1
  startstop prototype/1(CMD_ICE_ENABLE) -> Logical Operator/1
  CMD_ENERGY_MANAGER/1 -> Logical Operator/2
  Logical Operator/1 -> Data Type Conversion/1
  START/1 -> START/STOP 1/1(START)
  Delay3/1 -> startstop prototype/3(START_STOP_ENABLE)
  Data Type Conversion/1 -> START/STOP 1/2(CMD_START_STOP)
  START/STOP 1/1(FA_START_ICE) -> FA_START_ICE/1

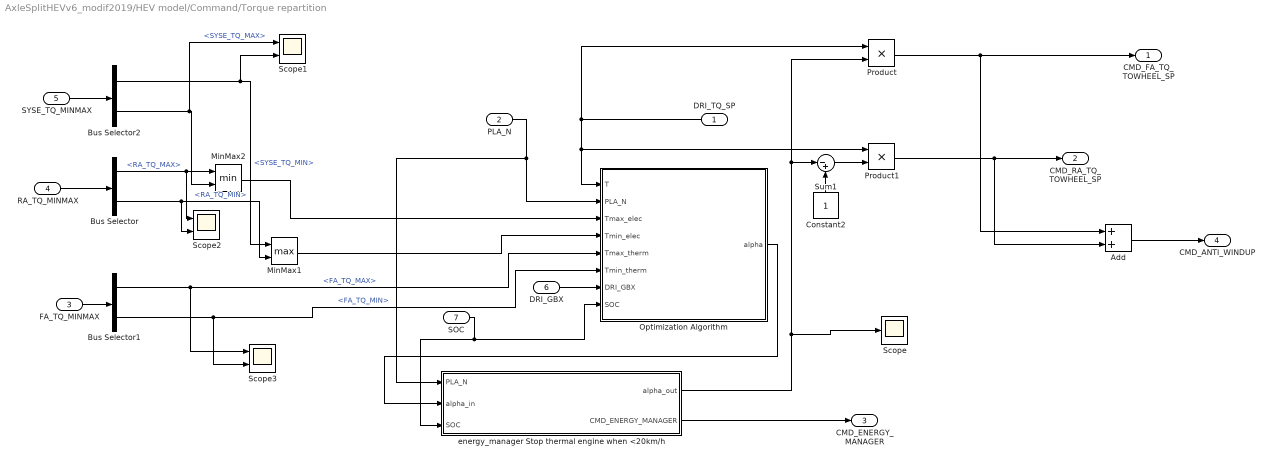
== system AxleSplitHEVv6_modif2019/HEV model/Command/Torque repartition ==
  DRI_TQ_SP : Inport
  PLA_N : Inport  Port=2
  FA_TQ_MINMAX : Inport  Port=3
  RA_TQ_MINMAX : Inport  Port=4
  SYSE_TQ_MINMAX : Inport  Port=5
  DRI_GBX : Inport  Port=6
  SOC : Inport  Port=7
  Add : Sum
  Bus Selector : BusSelector  OutputSignals=RA_TQ_MAX,RA_TQ_MIN
  Bus Selector1 : BusSelector  OutputSignals=FA_TQ_MAX,FA_TQ_MIN
  Bus Selector2 : BusSelector  OutputSignals=SYSE_TQ_MIN,SYSE_TQ_MAX
  Constant2 : Constant
  MinMax1 : MinMax  Function=max  Inputs=2  SampleTime=hev_dt
  MinMax2 : MinMax  Inputs=2  SampleTime=hev_dt
  "Optimization Algorithm " : Subsystem
  Product : Product
  Product1 : Product
  Scope : Scope
  Scope1 : Scope  NumInputPorts=2
  Scope2 : Scope  NumInputPorts=2
  Scope3 : Scope  NumInputPorts=2
  Sum1 : Sum  Inputs=|-+
  energy_manager Stop thermal engine when <20km/h : Subsystem
  CMD_FA_TQ_TOWHEEL_SP : Outport
  CMD_RA_TQ_TOWHEEL_SP : Outport  Port=2
  CMD_ENERGY_MANAGER : Outport  Port=3
  CMD_ANTI_WINDUP : Outport  Port=4
  wires:
  Product1/1 -> Add/2, CMD_RA_TQ_TOWHEEL_SP/1
  PLA_N/1 -> "Optimization Algorithm "/2(PLA_N), energy_manager Stop thermal engine when <20km/h/1(PLA_N)
  Sum1/1 -> Product1/2
  MinMax2/1 -> "Optimization Algorithm "/3(Tmax_elec)
  MinMax1/1 -> "Optimization Algorithm "/4(Tmin_elec)
  Constant2/1 -> Sum1/2
  RA_TQ_MINMAX/1 -> Bus Selector/1
  SYSE_TQ_MINMAX/1 -> Bus Selector2/1
  Bus Selector2/1 -> Scope1/2, MinMax1/1  "<SYSE_TQ_MIN>"
  Bus Selector/2 -> Scope2/2, MinMax1/2  "<RA_TQ_MIN>"
  Bus Selector/1 -> Scope2/1, MinMax2/1  "<RA_TQ_MAX>"
  Bus Selector2/2 -> Scope1/1, MinMax2/2  "<SYSE_TQ_MAX>"
  FA_TQ_MINMAX/1 -> Bus Selector1/1
  DRI_GBX/1 -> "Optimization Algorithm "/7(DRI_GBX)
  Bus Selector1/1 -> Scope3/1, "Optimization Algorithm "/5(Tmax_therm)  "<FA_TQ_MAX>"
  Bus Selector1/2 -> Scope3/2, "Optimization Algorithm "/6(Tmin_therm)  "<FA_TQ_MIN>"
  DRI_TQ_SP/1 -> Product1/1, "Optimization Algorithm "/1(T), Product/1
  SOC/1 -> "Optimization Algorithm "/8("SOC "), energy_manager Stop thermal engine when <20km/h/3(SOC)
  energy_manager Stop thermal engine when <20km/h/1(alpha_out) -> Scope/1, Product/2, Sum1/1
  "Optimization Algorithm "/1(alpha) -> energy_manager Stop thermal engine when <20km/h/2(alpha_in)
  energy_manager Stop thermal engine when <20km/h/2(CMD_ENERGY_MANAGER) -> CMD_ENERGY_MANAGER/1
  Product/1 -> Add/1, CMD_FA_TQ_TOWHEEL_SP/1
  Add/1 -> CMD_ANTI_WINDUP/1

== system AxleSplitHEVv6_modif2019/HEV model/Driver1/Clutch command ==
  note: On omet ce block
  DRI_REF_GBX : Inport
  FA_N_ICE : Inport  Port=2
  Clutch Command : Subsystem
  Clutch Stuck : Subsystem
  Terminator : Terminator
  DRI_GBX_SP : Outport
  DRI_CLUTCH_SP : Outport  Port=2
  wires:
  DRI_REF_GBX/1 -> Clutch Command/1(DRI_REF_GBX), Clutch Stuck/1(REF_GBX)
  Clutch Command/2(DRI_GBX_SP) -> DRI_GBX_SP/1
  FA_N_ICE/1 -> Clutch Stuck/2(FA_N_ICE)
  Clutch Command/1(DRI_CLUTCH_SP) -> DRI_CLUTCH_SP/1, Clutch Stuck/3(DRI_CLU_SP)
  Clutch Stuck/1(OUT_CLU) -> Terminator/1

== system AxleSplitHEVv6_modif2019/HEV model/Driver1/Doc Driver ==

== system AxleSplitHEVv6_modif2019/HEV model/Driver1/Driver ==
  CMD_ANTI_WINDUP : Inport
  DRI_DELTA_SPEED : Inport  Port=2
  Compare To Constant : simulink/Logic and Bit Operations/Compare To Constant  relop=<=  const=200  OutDataTypeStr=uint8
  Discrete Zero-Pole : DiscreteZeroPole  Zeros=[-1]  Poles=[1]  Gain=1  SampleTime=hev_dt
  FA_N_ICE : InportShadow  Port=2
  Gain1 : Gain  Gain=dri_ki/dri_kp  SampleTime=hev_dt
  Gain2 : Gain  Gain=-1
  Gain4 : Gain  Gain=dri_ki  SampleTime=hev_dt
  Gain5 : Gain  Gain=dri_kp  SampleTime=hev_dt
  Gain7 : Gain  Gain=hev_dt/2  SampleTime=hev_dt
  Ground : Ground
  Saturation : Saturate  UpperLimit=inf  LowerLimit=0
  Saturation1 : Saturate  UpperLimit=0  LowerLimit=-inf
  Sum1 : Sum  Inputs=++|  SampleTime=hev_dt
  Sum2 : Sum  Inputs=|++  SampleTime=hev_dt
  Terminator1 : Terminator
  DRI_TQ_SP : Outport
  CMD_BRAKE : Outport  Port=2
  DRI_CLUTCH : Outport  Port=3
  wires:
  Gain5/1 -> Sum2/2
  Gain4/1 -> Sum1/2
  Sum1/1 -> Gain7/1
  Discrete Zero-Pole/1 -> Sum2/1
  CMD_ANTI_WINDUP/1 -> Gain1/1
  DRI_DELTA_SPEED/1 -> Gain5/1, Gain4/1
  Sum2/1 -> Saturation1/1, Saturation/1
  Gain7/1 -> Discrete Zero-Pole/1
  Saturation/1 -> DRI_TQ_SP/1
  Saturation1/1 -> Gain2/1
  Ground/1 -> Terminator1/1
  Gain1/1 -> Sum1/1
  Gain2/1 -> CMD_BRAKE/1
  FA_N_ICE/1 -> Compare To Constant/1
  Compare To Constant/1 -> DRI_CLUTCH/1

== system AxleSplitHEVv6_modif2019/HEV model/Electrical system/Auxiliary network 12V ==
  SYSE_VOLTAGE_HV : Inport
  Auxliliary network : Subsystem
  CVS : Subsystem
  SYSE_AUX_CURRENT : Outport
  wires:
  Auxliliary network/1(SYSE_CURRENT_LV) -> CVS/1(SYSE_CURRENT_LV)
  Auxliliary network/2(SYSE_VOLTAGE_LV) -> CVS/2(SYSE_VOLTAGE_LV)
  CVS/1(SYSE_AUX_CURRENT) -> SYSE_AUX_CURRENT/1
  SYSE_VOLTAGE_HV/1 -> CVS/3(SYSE_VOLTAGE_HV)

== system AxleSplitHEVv6_modif2019/HEV model/Electrical system/Doc Electrical system ==

== system AxleSplitHEVv6_modif2019/HEV model/Electrical system/Electrical System supervision ==
  RA_N_EM : Inport
  SYSE_SOC : Inport  Port=2
  SYSE_AUX_CURRENT : Inport  Port=3
  SYSE_VOLTAGE_HV : Inport  Port=4
  DRI_GBX_SP : Inport  Port=5
  Battery charge / discharge limits : Subsystem
  Current loop : Subsystem
  Demux : Demux  Outputs=2
  "Min max " : Subsystem
  Mux : Mux  Inputs=2
  Torque conversion : Subsystem
  SYSE_TQ_MAX : Outport
  SYSE_TQ_MIN : Outport  Port=2
  wires:
  SYSE_SOC/1 -> Battery charge / discharge limits/1(SYSE_SOC)
  Battery charge / discharge limits/1(SYSE_I_DISCHARGE) -> Current loop/2(SYSE_I_DISCHARGE)  "A"
  Battery charge / discharge limits/2(SYSE_I_CHARGE) -> Current loop/3(SYSE_I_CHARGE)  "A"
  Current loop/1(SYSE_EM_I_DISCHARGE) -> "Min max "/1(SYSE_EM_I_DISCHARGE)
  Current loop/2(SYSE_EM_I_CHARGE) -> "Min max "/2(SYSE_EM_I_CHARGE)
  SYSE_AUX_CURRENT/1 -> Current loop/1(SYSE_AUX_CURRENT)  "A"
  SYSE_VOLTAGE_HV/1 -> "Min max "/3(SYSE_VOLTAGE_HV)  "V"
  RA_N_EM/1 -> "Min max "/4(PLA_N_EM), Torque conversion/2(RA_N_EM)
  "Min max "/2(SYSE_TQ_MIN_BMS) -> Mux/2
  "Min max "/1(SYSE_TQ_MAX_BMS) -> Mux/1
  Torque conversion/1(SYSE_TQ_MINMAX) -> Demux/1
  Demux/2 -> SYSE_TQ_MIN/1
  Demux/1 -> SYSE_TQ_MAX/1
  Mux/1 -> Torque conversion/1(SYSE_TQ_MINMAX_BMS)
  DRI_GBX_SP/1 -> Torque conversion/3(DRI_GBX_SP)

== system AxleSplitHEVv6_modif2019/HEV model/Electrical system/Lithium-Ion Battery Management System ==
  note: Convention:
      | Positive current -> discharge
      | Negative current -> charge
  SYSE_LIION_CURRENT : Inport
  Battery control : Subsystem
  Battery model : Subsystem
  Battery power contactor : Subsystem
  Delay : Delay  DelayLength=1  SampleTime=hev_dt
  SYSE_SOC : Outport
  SYSE_VOLTAGE_HV : Outport  Port=2
  wires:
  SYSE_LIION_CURRENT/1 -> Battery control/1(SYSE_LIION_CURRENT), Battery power contactor/2(SYSE_LIION_CURRENT)  "A"
  Battery model/2(SYSE_SOC) -> SYSE_SOC/1, Delay/1
  Battery model/1(SYSE_VOLTAGE_HV) -> SYSE_VOLTAGE_HV/1
  Battery control/1(SYSE_LIION_CONTACTOR_OPEN_REQ) -> Battery power contactor/1(SYSE_LIION_CONTACTOR_OPEN_REQ)  "[-]"
  Battery power contactor/1(SYSE_LIION_CURRENT_OUT) -> Battery model/1(SYSE_LIION_CURRENT_OUT)
  Delay/1 -> Battery control/2(SYSE_SOC)

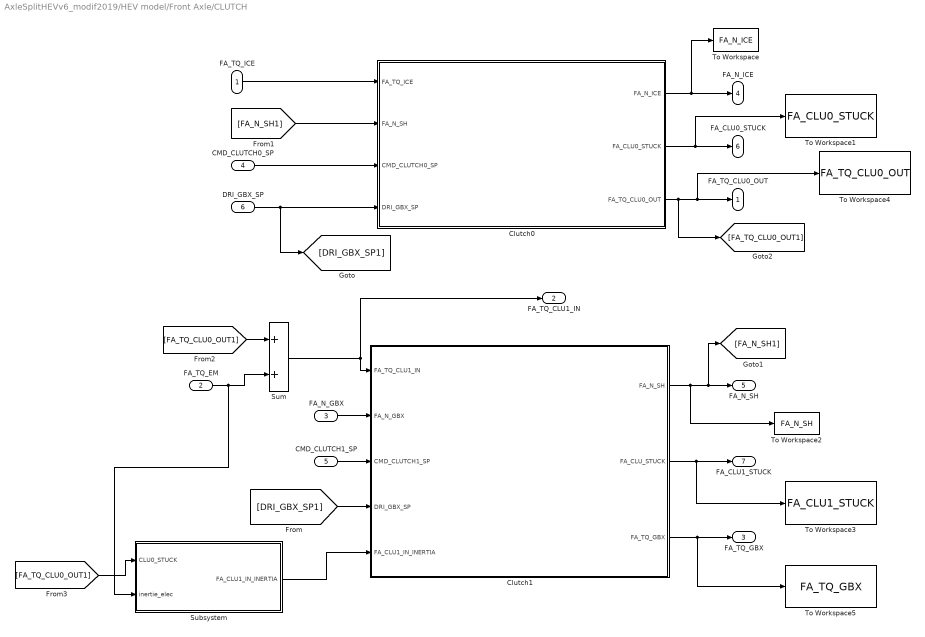
== system AxleSplitHEVv6_modif2019/HEV model/Front Axle/CLUTCH ==
  FA_TQ_ICE : Inport
  FA_TQ_EM : Inport  Port=2
  FA_N_GBX : Inport  Port=3
  CMD_CLUTCH0_SP : Inport  Port=4
  CMD_CLUTCH1_SP : Inport  Port=5
  DRI_GBX_SP : Inport  Port=6
  Clutch0 : Subsystem
  Clutch1 : Subsystem
  Subsystem : Subsystem
  Sum : Sum
  To Workspace : ToWorkspace  VariableName=FA_N_ICE  SampleTime=-1
  To Workspace1 : ToWorkspace  VariableName=FA_CLU0_STUCK  SampleTime=-1
  To Workspace2 : ToWorkspace  VariableName=FA_N_SH  SampleTime=-1
  To Workspace3 : ToWorkspace  VariableName=FA_CLU1_STUCK  SampleTime=-1
  To Workspace4 : ToWorkspace  VariableName=FA_TQ_CLU0_OUT  SampleTime=-1
  To Workspace5 : ToWorkspace  VariableName=FA_TQ_GBX  SampleTime=-1
  FA_TQ_CLU0_OUT : Outport
  FA_TQ_CLU1_IN : Outport  Port=2
  FA_TQ_GBX : Outport  Port=3
  FA_N_ICE : Outport  Port=4
  FA_N_SH : Outport  Port=5
  FA_CLU0_STUCK : Outport  Port=6
  FA_CLU1_STUCK : Outport  Port=7
  wires:
  Clutch0/1(FA_N_ICE) -> To Workspace/1, FA_N_ICE/1
  DRI_GBX_SP/1 -> [DRI_GBX_SP1], Clutch0/4(DRI_GBX_SP)
  CMD_CLUTCH0_SP/1 -> Clutch0/3(CMD_CLUTCH0_SP)
  FA_TQ_ICE/1 -> Clutch0/1(FA_TQ_ICE)
  Clutch0/2(FA_CLU0_STUCK) -> To Workspace1/1, FA_CLU0_STUCK/1
  [FA_N_SH1] -> Clutch0/2(FA_N_SH)
  [DRI_GBX_SP1] -> Clutch1/4(DRI_GBX_SP)
  CMD_CLUTCH1_SP/1 -> Clutch1/3(CMD_CLUTCH1_SP)
  FA_N_GBX/1 -> Clutch1/2(FA_N_GBX)
  Sum/1 -> Clutch1/1(FA_TQ_CLU1_IN), FA_TQ_CLU1_IN/1
  Clutch0/3(FA_TQ_CLU0_OUT) -> [FA_TQ_CLU0_OUT1], To Workspace4/1, FA_TQ_CLU0_OUT/1
  [FA_TQ_CLU0_OUT1] -> Sum/1
  Clutch1/2(FA_CLU_STUCK) -> To Workspace3/1, FA_CLU1_STUCK/1
  Clutch1/1(FA_N_SH) -> To Workspace2/1, [FA_N_SH1], FA_N_SH/1
  Clutch1/3(FA_TQ_GBX) -> To Workspace5/1, FA_TQ_GBX/1
  Subsystem/1(FA_CLU1_IN_INERTIA) -> Clutch1/5(FA_CLU1_IN_INERTIA)
  [FA_TQ_CLU0_OUT1] -> Subsystem/1(CLU0_STUCK)
  FA_TQ_EM/1 -> Subsystem/2("inertie_elec "), Sum/2

== system AxleSplitHEVv6_modif2019/HEV model/Front Axle/Doc Front axle ==

== system AxleSplitHEVv6_modif2019/HEV model/Front Axle/Electrical machine ==
  CMD_FA_TQ_ICE_SP : Inport
  FA_N_EM : Inport  Port=2
  SYSE_VOLTAGE_HV : Inport  Port=3
  Divide1 : Product  Inputs=*/  SampleTime=hev_dt
  Engine representation : Subsystem
  Power efficiency : Subsystem
  FA_EM_CURRENT : Outport
  FA_TQ_EM : Outport  Port=2
  FA_TQ_MIN_EM : Outport  Port=3
  FA_TQ_MAX_EM : Outport  Port=4
  wires:
  Engine representation/1(FA_TQ_EM) -> FA_TQ_EM/1, Power efficiency/1(FA_TQ_EM)
  CMD_FA_TQ_ICE_SP/1 -> Engine representation/1(CMD_FA_TQ_ICE_SP)
  FA_N_EM/1 -> Engine representation/2(FA_N_EM), Power efficiency/2(FA_N_EM)
  Engine representation/2(FA_TQ_MIN_EM) -> FA_TQ_MIN_EM/1
  Engine representation/3(FA_TQ_MAX_EM) -> FA_TQ_MAX_EM/1
  Power efficiency/1(RA_EM_POWER) -> Divide1/1
  SYSE_VOLTAGE_HV/1 -> Divide1/2
  Divide1/1 -> FA_EM_CURRENT/1

== system AxleSplitHEVv6_modif2019/HEV model/Front Axle/FA_TQ_to_F_BRAKE ==
  CMD_FA_MECANICAL_BRAKE : Inport
  Gain : Gain  Gain=1/pla_wheel_radius
  FA_PLA_F_BRAKE : Outport
  wires:
  CMD_FA_MECANICAL_BRAKE/1 -> Gain/1
  Gain/1 -> FA_PLA_F_BRAKE/1

== system AxleSplitHEVv6_modif2019/HEV model/Front Axle/ICE ==
  CMD_FA_TQ_SP : Inport
  FA_ICE_RESET_SYNCHRO : Inport  Port=2
  FA_START_ICE : Inport  Port=3
  DRI_GBX_SP : Inport  Port=4
  FA_CLU_STUCK : Inport  Port=5
  FA_N_ICE : Inport  Port=6
  ICE : Subsystem
  ICE control : Subsystem
  FA_ICE_STATE : Outport
  FA_GAS_CONSUMPTION : Outport  Port=2
  FA_TQ_MAX_ICE : Outport  Port=3
  FA_TQ_MIN_ICE : Outport  Port=4
  FA_TQ_ICE : Outport  Port=5
  wires:
  ICE/1(FA_GAS_CONSUMPTION) -> FA_GAS_CONSUMPTION/1
  ICE/2(FA_TQ_ICE) -> FA_TQ_ICE/1
  ICE control/2(FA_ICE_TQ_SP) -> ICE/2(FA_ICE_TQ_SP)
  CMD_FA_TQ_SP/1 -> ICE control/2(CMD_FA_TQ_ICE_SP)
  ICE control/1(FA_TQ_MAX_ICE) -> FA_TQ_MAX_ICE/1
  FA_N_ICE/1 -> ICE/1(FA_N_ICE), ICE control/1(FA_N_ICE)
  DRI_GBX_SP/1 -> ICE control/3(DRI_GBX_SP)
  ICE control/3(FA_STARTER_REQUEST) -> ICE/3(FA_STARTER_REQUEST)
  FA_CLU_STUCK/1 -> ICE control/4(FA_CLU_STUCK)
  FA_START_ICE/1 -> ICE control/5(FA_START_ICE)
  ICE control/5(FA_TQ_MIN_ICE) -> FA_TQ_MIN_ICE/1
  ICE control/4(FA_ICE_STATE) -> FA_ICE_STATE/1, ICE/4(FA_ICE_STATE)
  FA_ICE_RESET_SYNCHRO/1 -> ICE control/6(FA_ICE_RESET_SYNCHRO)
  ICE/3(FA_TQ_STARTER) -> ICE control/7(FA_TQ_STARTER)

== system AxleSplitHEVv6_modif2019/HEV model/Front Axle/Reducteur ==
  FA_TQ_&_MINMAX_EM : Inport
  FA_N_SH : Inport  Port=2
  Differential ratio : Gain  Gain=reducteur  SampleTime=hev_dt
  Divide1 : Product  SampleTime=hev_dt
  Efficiency P neg : Gain  Gain=2-ra_transmission_efficiency  SampleTime=hev_dt
  Efficiency P pos : Gain  Gain=ra_transmission_efficiency  SampleTime=hev_dt
  Switch : Switch  SampleTime=hev_dt
  differential ratio : Gain  Gain=reducteur  SampleTime=hev_dt
  FA_TQ_&_MINMAX_EM_SH : Outport
  FA_N_EM : Outport  Port=2
  wires:
  FA_TQ_&_MINMAX_EM/1 -> Divide1/2, Efficiency P neg/1, Efficiency P pos/1
  Efficiency P pos/1 -> Switch/1
  Efficiency P neg/1 -> Switch/3
  Divide1/1 -> Switch/2
  Switch/1 -> Differential ratio/1
  FA_N_SH/1 -> Divide1/1, differential ratio/1
  Differential ratio/1 -> FA_TQ_&_MINMAX_EM_SH/1
  differential ratio/1 -> FA_N_EM/1
